simulink model "Sys1t"  (Simulink 7.8)
settings: Solver=ode45  StartTime=0.0  StopTime=time_span  RelTol=1e-3
undefined symbols (not defined in the file): noise_on, samp_time, Td, Ti, Tk
libraries: simulink x1, simulink_need_slupdate x1
settings Model: Creator=Jim  LastModifiedBy=TheQuarry
settings DataIOCC: LimitDataPoints=off  SaveTime=off  TimeSaveName=t
settings OptimizationCC: InitFltsAndDblsToZero=on
settings DebuggingCC: SaveWithParameterizedLinksMsg=none  FcnCallInpInsideContextMsg=Use local settings  StrictBusMsg=Warning
settings GRTTargetCC: TargetFcnLib=ansi_tfl_tmw.mat

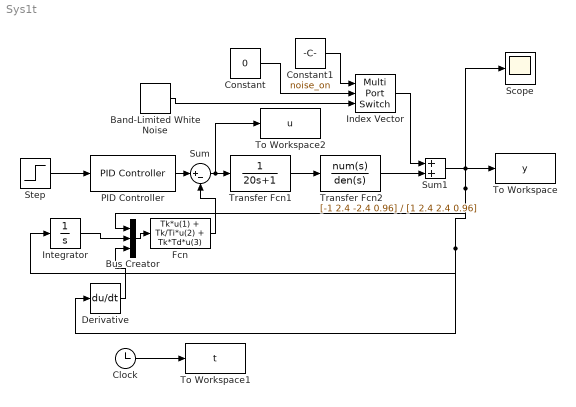
== system Sys1t ==
  Band-Limited White Noise : simulink/Sources/Band-Limited White Noise  Cov=[0.0001]  Ts=0.1  seed=[23341]
  Bus Creator : BusCreator  Inputs=3
  Clock : Clock
  Constant : Constant  Value=0
  Constant1 : Constant  Value=noise_on
  Derivative : Derivative
  Fcn : Fcn  Expr=Tk*u(1) + Tk/Ti*u(2) + Tk*Td*u(3)
  Index Vector : MultiPortSwitch  DataPortOrder=Zero-based contiguous  Inputs=2  zeroidx=on
  Integrator : Integrator
  PID Controller : simulink_need_slupdate/PID Controller  P=Tk  I=Tk/Ti  D=0
  Scope : Scope
  Step : Step  Time=0  SampleTime=0
  Sum : Sum  Inputs=|+-
  Sum1 : Sum  Inputs=|++
  To Workspace : ToWorkspace  VariableName=y  SampleTime=samp_time  SaveFormat=Array
  To Workspace1 : ToWorkspace  VariableName=t  SampleTime=samp_time  SaveFormat=Array
  To Workspace2 : ToWorkspace  VariableName=u  SampleTime=samp_time  SaveFormat=Array
  Transfer Fcn1 : TransferFcn  Denominator=[20 1]
  Transfer Fcn2 : TransferFcn  Numerator="[-1\t2.4\t-2.4\t0.96]"  Denominator="[1\t2.4\t2.4\t0.96]"
  wires:
  Sum/1 -> Transfer Fcn1/1, To Workspace2/1
  Sum1/1 -> To Workspace/1, Scope/1, Bus Creator/1, Derivative/1, Integrator/1
  Step/1 -> PID Controller/1
  PID Controller/1 -> Sum/1
  Transfer Fcn2/1 -> Sum1/2
  Transfer Fcn1/1 -> Transfer Fcn2/1
  Index Vector/1 -> Sum1/1
  Constant1/1 -> Index Vector/1
  Constant/1 -> Index Vector/2
  Band-Limited White Noise/1 -> Index Vector/3
  Clock/1 -> To Workspace1/1
  Fcn/1 -> Sum/2
  Bus Creator/1 -> Fcn/1
  Integrator/1 -> Bus Creator/2
  Derivative/1 -> Bus Creator/3
